simulink model "Robust_RotPen_2021b"  (R2021b)
settings: Solver=VariableStepAuto  StartTime=0.0  StopTime=10  RelTol=1e-3
libraries: cstblocks x1
settings Model: Creator=djangovanderplas  LastModifiedBy=thoma
settings DebuggingCC: UnconnectedInputMsg=none  UnconnectedOutputMsg=none  UnconnectedLineMsg=none
settings ModelReferenceCC: EnableRefExpFcnMdlSchedulingChecks=off
settings RTWCC: GPUComputeCapability=5.0  DLArmComputeVersion=20.02.1
settings ConfigComp: CovBoundaryAbsTol=1.0e-5

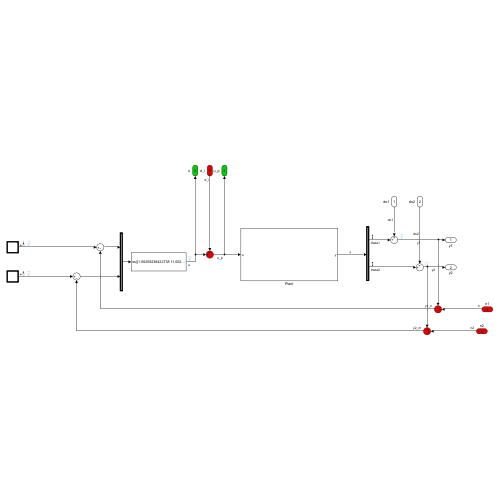
[thumbnail: Simulink's stored preview of the top-level diagram]
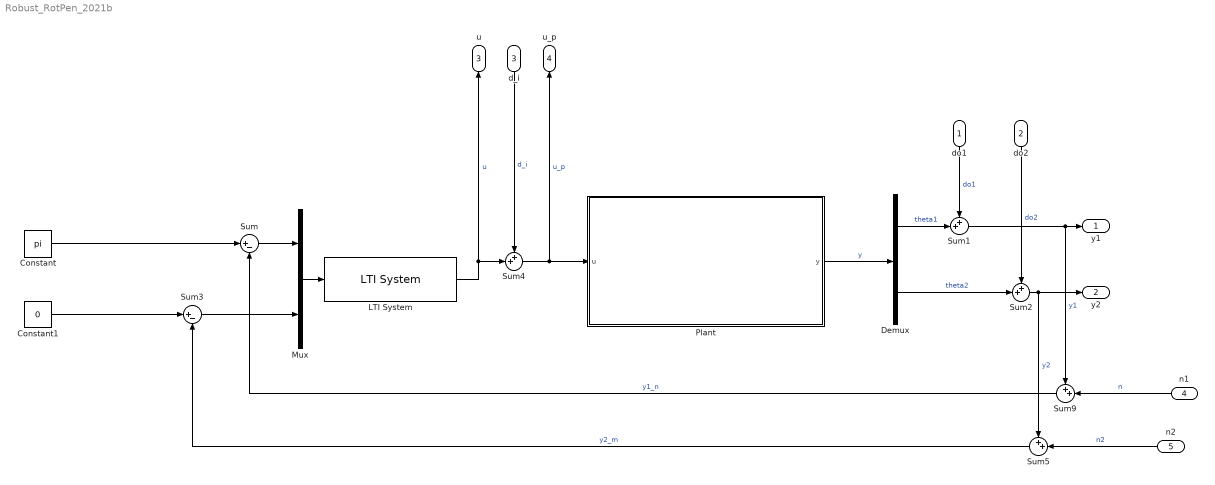
== system Robust_RotPen_2021b ==
  do1 : Inport  PortDimensions=1
  do2 : Inport  Port=2  PortDimensions=1
  d_i : Inport  Port=3
  n1 : Inport  Port=4  PortDimensions=1
  n2 : Inport  Port=5  PortDimensions=1
  Constant : Constant  Value=pi
  Constant1 : Constant  Value=0
  Demux : Demux  Outputs=2
  LTI System : cstblocks/LTI System  sys=ss([1.06259238422738 11.0024393047227 0 0;0.226679408218701 -5.79388949545269 -13.2487025243059 0;0 -1.45003484090123 -2.14585259544542 -3.32009142788137;0 0 10.8781045181047 -6.27471667499045],[4.96303389878086 -16.4610222766717;-2.43738277274122 8.72178947964596;-1.5270052509986 1.49360410486402;2.1440025642701 -3.80757417672494],[0.18090788254952 0.233134934718946 -3.41053695053143 0.600213790753142],[0.0261701634839277 -0.0261701634839277],0)  IC=[]
  Mux : Mux  Inputs=2
  Plant : Subsystem
  Sum : Sum  Inputs=|+-
  Sum{1..2,4..5,9} (5 alike) : Sum  Inputs=++|
  Sum3 : Sum  Inputs=|+-
  y1 : Outport  PortDimensions=1
  y2 : Outport  Port=2  PortDimensions=1
  u : Outport  Port=3
  u_p : Outport  Port=4
  wires:
  Plant/1(y) -> Demux/1  "y"
  Constant/1 -> Sum/1
  Demux/2 -> Sum2/2  "theta2"
  Demux/1 -> Sum1/2  "theta1"
  do1/1 -> Sum1/1  "do1"
  do2/1 -> Sum2/1  "do2"
  Sum1/1 -> y1/1, Sum9/1  "y1"
  Sum2/1 -> Sum5/1, y2/1  "y2"
  LTI System/1 -> u/1, Sum4/2  "u"
  d_i/1 -> Sum4/1  "d_i"
  Sum4/1 -> Plant/1(u), u_p/1  "u_p"
  n1/1 -> Sum9/2  "n"
  n2/1 -> Sum5/2  "n2"
  Sum9/1 -> Sum/2  "y1_n"
  Sum5/1 -> Sum3/2  "y2_m"
  Constant1/1 -> Sum3/1
  Mux/1 -> LTI System/1
  Sum3/1 -> Mux/2
  Sum/1 -> Mux/1

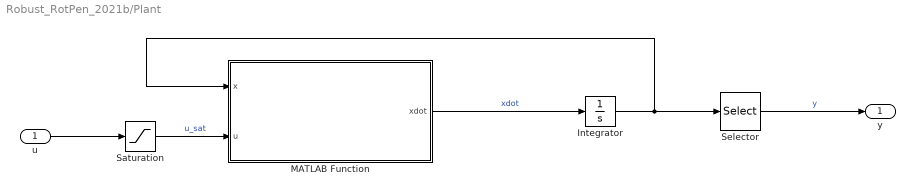
== system Robust_RotPen_2021b/Plant ==
  u : Inport
  Integrator : Integrator  InitialCondition=[pi+0.2;-0.1;0;0]
  MATLAB Function : MATLAB Function  TreatAsAtomicUnit=on
  Saturation : Saturate  UpperLimit=1  LowerLimit=-1
  Selector : Selector  InputPortWidth=4  IndexOptions=Index vector (dialog)  Indices=[1 2]  OutputSizes=1
  y : Outport
  wires:
  Selector/1 -> y/1  "y"
  Integrator/1 -> Selector/1, MATLAB Function/1(x)
  MATLAB Function/1(xdot) -> Integrator/1  "xdot"
  u/1 -> Saturation/1
  Saturation/1 -> MATLAB Function/2(u)  "u_sat"

== matlab function Robust_RotPen_2021b/Plant/MATLAB Function ==
  data: x input; u input; xdot output
function xdot = nonlinearPlant(x,u)

% State vector
theta1  = x(1);
theta2  = x(2);
dtheta1 = x(3);
dtheta2 = x(4);

% ============================================================
% Parameters
% ============================================================

pa       = 64.7915;
pb1      = 3.2117e3;
pc1      = 635.3865;
pg1      = 430.5226;
pu       = 2.2424e4;
p0       = 0;

pb2      = 0.0670;
pg2      = 112.0268;
pc2      = 0.2491;
psdelta2 = 0.1836;

epsv1    = 0.05;
epsv2    = 0.03;
vs2      = 3.5;

l1 = 0.1;
g  = 9.81;
pc = (l1/g)*pg2;

% ============================================================
% Dynamics
% ============================================================

c2 = cos(theta2);
s2 = sin(theta2);

% Inertia matrix
M11 = pa + 1 + 2*pc*c2;
M12 = 1 + pc*c2;
M21 = M12;
M22 = 1;

% Coriolis/Centrifugal terms
Cqdot1 = -pc*s2*(2*dtheta1*dtheta2 + dtheta2^2);
Cqdot2 =  pc*s2*dtheta1^2;

% Friction
F1 = pb1*dtheta1 + pc1*tanh(dtheta1/epsv1);

stribeck2 = pc2 + psdelta2*exp(-(dtheta2/vs2)^2);
F2 = pb2*dtheta2 + stribeck2*tanh(dtheta2/epsv2);

% Gravity
G1 = -pg1*sin(theta1) - pg2*sin(theta1 + theta2);
G2 = -pg2*sin(theta1 + theta2);

% Input torques
I1 = pu*u + p0;
I2 = 0;

% Right-hand side
rhs1 = I1 - Cqdot1 - F1 - G1;
rhs2 = I2 - Cqdot2 - F2 - G2;

% Solve M*qdd = rhs
detM = M11*M22 - M12*M21;

ddtheta1 = ( M22*rhs1 - M12*rhs2)/detM;
ddtheta2 = (-M21*rhs1 + M11*rhs2)/detM;

% State derivative
xdot = zeros(4,1);

xdot(1) = dtheta1;
xdot(2) = dtheta2;
xdot(3) = ddtheta1;
xdot(4) = ddtheta2;

end
